simulink model "L4_6"  (R2023a)
settings: Solver=VariableStepAuto  StartTime=0.0  StopTime=160  RelTol=1e-15
settings Model: Creator=apere  LastModifiedBy=apere

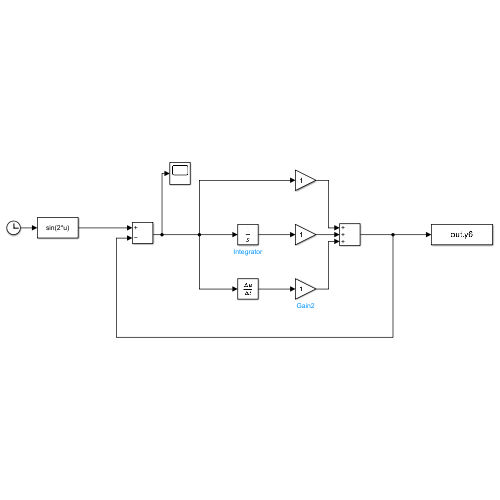
[thumbnail: Simulink's stored preview of the top-level diagram]
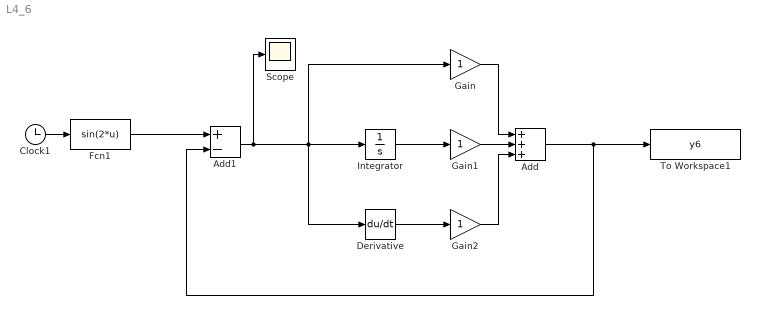
== system L4_6 ==
  Add : Sum  Inputs=+++
  Add1 : Sum  Inputs=+-
  Clock1 : Clock
  Derivative : Derivative
  Fcn1 : Fcn  Expr=sin(2*u)
  Gain : Gain
  Gain1 : Gain
  Gain2 : Gain
  Integrator : Integrator
  Scope : Scope
  To Workspace1 : ToWorkspace  VariableName=y6  SaveFormat=Timeseries  SampleTime=-1
  wires:
  Clock1/1 -> Fcn1/1
  Fcn1/1 -> Add1/1
  Add1/1 -> Derivative/1, Gain/1, Integrator/1, Scope/1
  Add/1 -> Add1/2, To Workspace1/1
  Gain/1 -> Add/1
  Gain1/1 -> Add/2
  Gain2/1 -> Add/3
  Integrator/1 -> Gain1/1
  Derivative/1 -> Gain2/1
